simulink library "lights"  (Simulink 7.6)
settings: Solver=ode45  SolverMode=SingleTasking  StartTime=0.0  StopTime=10.0  RelTol=1e-3
settings Model: Creator=The MathWorks Inc.

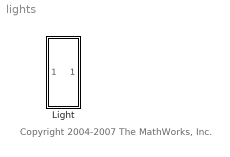
== system lights ==
  note: Copyright 2004-2007 The MathWorks, Inc.
  Light : Subsystem  mask(Light){state=Stop}
      mask help: Place this light block on a boolean signal and it will indicate the signal's value as green when it is true, and red when false. Non-boolean signals are treated as false if equal to zero, and true otherwise. Note that the input signal is passed straight through to the output of this block. For signals that are connected to trigger ports, an automatic delay of 50 ms is added when the trigger fires.
      mask init:
      | s = get_param(gcbh, 'position'); w = s(3)-s(1);h = s(4)-s(2);
      | r = min(w, h/2)/2;ang = 0:0.1:2*pi;
      | x1 = r*sin(ang)+w/2; y1 = r*cos(ang)+0.75*h;
      | x2 = r*sin(ang)+w/2; y2 = r*cos(ang)+0.25*h;
      | 
      | if strcmp(state,'Stop')
      |  c1 = [1 0 0]; c2 = [0 0 0];
      | else
      |  c1 = [0 0 0]; c2 = [0 1 0];
      | end
      mask StyleString: popup(Stop|Go)
      mask Display:
      | patch([0 w w 0],[h h 0 0],[0.7 0.7, 0.7])
      | patch(x1,y1,c1)
      | patch(x2,y2,c2)

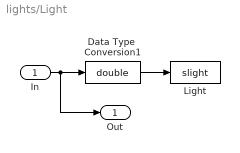
== system lights/Light ==
  In : Inport
  Data Type  Conversion1 : DataTypeConversion  OutDataTypeStr=double  SaturateOnIntegerOverflow=on  RndMeth=Zero
  Light : S-Function  FunctionName=slight  EnableBusSupport=off
  Out : Outport
  wires:
  Data Type  Conversion1/1 -> Light/1
  In/1 -> Data Type  Conversion1/1, Out/1
